simulink model "CSRT_NL"  (R2020b)
settings: Solver=FixedStepAuto  StartTime=0.0  StopTime=15  FixedStep=0.01  RelTol=1e-3
values from neighbouring files (symbols this model uses):
  Cafs = 10    [CSTR_PID.m]
  Cas = 8.564    [CSTR_PID.m]
  dCafs = 0    [CSTR_PID.m]
  dTfs = 0    [CSTR_PID.m]
  dTjs = 0    [CSTR_PID.m]
  Fs = 1    [CSTR_PID.m]
  Ki1 = Kp1/Ti1    (= 18.4487621431)    [CSTR_PID.m]
  Kp1 = (T/(K*L))*(0.9 + L/(12*T))    (= 5.91300687974)    [CSTR_PID.m]    (also in Exp2_guia.m = 0.469047619048)
  RefCa = 9    [CSTR_PID.m]
  Tfs = 298    [CSTR_PID.m]
  Tjs = 298    [CSTR_PID.m]
  Ts = 311.2    [CSTR_PID.m]
libraries: pid_lib x1
settings Model: Creator=franc  LastModifiedBy=Francinildo Barbosa

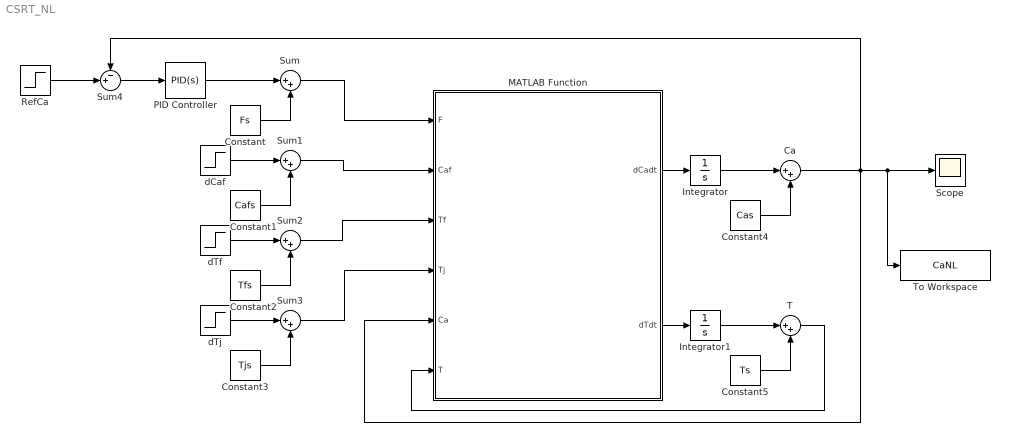
== system CSRT_NL ==
  "              Ca" : Sum  Inputs=|++
  "            T" : Sum  Inputs=|++
  Constant : Constant  Value=Fs
  Constant1 : Constant  Value=Cafs
  Constant2 : Constant  Value=Tfs
  Constant3 : Constant  Value=Tjs
  Constant4 : Constant  Value=Cas
  Constant5 : Constant  Value=Ts
  Integrator : Integrator
  Integrator1 : Integrator
  MATLAB Function : MATLAB Function  TreatAsAtomicUnit=on
  PID Controller : pid_lib/PID Controller  Controller=PID  Form=Parallel  TimeDomain=Continuous-time  UseExternalTs=off  SampleTime=-1  IntegratorMethod=Forward Euler  FilterMethod=Forward Euler  ControllerParametersSource=internal  P=Kp1  I=Ki1  D=0  UseFilter=on  N=100  TunerSelectOption=Transfer Function Based (PID Tuner App)  InitialConditionSource=internal  InitialConditionForIntegrator=0  InitialConditionForFilter=0  DifferentiatorICPrevScaledInput=0  ExternalReset=none  TrackingMode=off  Kt=1  LimitOutput=off  SatLimitsSource=internal  UpperSaturationLimit=inf  LowerSaturationLimit=-inf  LinearizeAsGain=on  AntiWindupMode=none  Kb=1  POutMin=[]  POutMax=[]  IOutMin=[]  IOutMax=[]  DOutMin=[]  DOutMax=[]  NOutMin=[]  NOutMax=[]  SumOutMin=[]  SumOutMax=[]  SaturationOutMin=[]  SaturationOutMax=[]  PParamMin=[]  PParamMax=[]  IParamMin=[]  IParamMax=[]  DParamMin=[]  DParamMax=[]  NParamMin=[]  NParamMax=[]  KbParamMin=[]  KbParamMax=[]  KtParamMin=[]  KtParamMax=[]  KbOutMin=[]  KbOutMax=[]  KtOutMin=[]  KtOutMax=[]  IntegratorOutMin=[]  IntegratorOutMax=[]  FilterOutMin=[]  FilterOutMax=[]  SumI1OutMin=[]  SumI1OutMax=[]  SumI2OutMin=[]  SumI2OutMax=[]  SumI3OutMin=[]  SumI3OutMax=[]  SumI4OutMin=[]  SumI4OutMax=[]  SumDOutMin=[]  SumDOutMax=[]  DifferentiatorOutMin=[]  DifferentiatorOutMax=[]  FilterDiffOutCoefMin=[]  FilterDiffOutCoefMax=[]  ReciprocalOutMin=[]  ReciprocalOutMax=[]  SumDenOutMin=[]  SumDenOutMax=[]  SumNumOutMin=[]  SumNumOutMax=[]  DivideOutMin=[]  DivideOutMax=[]  UdiffTsProdOutMin=[]  UdiffTsProdOutMax=[]  NTsProdOutMin=[]  NTsProdOutMax=[]  UintegralTsProdOutMin=[]  UintegralTsProdOutMax=[]  UngainTsProdOutMin=[]  UngainTsProdOutMax=[]  IntegratorContinuousStateAttributes=''  IntegratorStateMustResolveToSignalObject=off  IntegratorRTWStateStorageClass=Auto  FilterContinuousStateAttributes=''  FilterStateMustResolveToSignalObject=off  FilterRTWStateStorageClass=Auto  ParallelPVariant=InternalParameters  IdealPVariant=Disabled  IVariant=InternalParameters  DVariant=InternalParameters  IntegratorVariant=Continuous  SatVariant=Disabled  AWVariant=Passthrough  PCopyVariant=Disabled  TRVariant=Disabled  FdbkBlocksVariant=Forward  IdealPFdbkVariant=Disabled  SatFdbkVariant=Disabled  DerivativeFilterVariant=ContFilter  NVariant=InternalParameters  NCopyVariant=Disabled  FilterICVariant=InternalICsFilter  IntegratorICVariant=InternalICs  ExternalResetVariant=Disabled  TRSumVariant=Passthrough  SumFdbkVariant=Disabled  SumVariant=Sum_PID  TsampFilterVariant=InternalTs  TsampNgainVariant=Passthrough  TsampIntegralVariant=Passthrough  ExternalSaturationOutDataTypeStr=Inherit: Same as second input
  RefCa : Step  Time=0  After=RefCa  SampleTime=0
  Scope : Scope
  Sum{,1..3} (4 alike) : Sum  Inputs=|++
  Sum4 : Sum  Inputs=-+|
  To Workspace : ToWorkspace  VariableName=CaNL  SaveFormat=Timeseries  SampleTime=-1
  dCaf : Step  Time=0  After=dCafs  SampleTime=0
  dTf : Step  Time=0  After=dTfs  SampleTime=0
  dTj : Step  Time=0  After=dTjs  SampleTime=0
  wires:
  Constant/1 -> Sum/2
  Sum/1 -> MATLAB Function/1(F)
  Constant1/1 -> Sum1/2
  dCaf/1 -> Sum1/1
  Sum1/1 -> MATLAB Function/2(Caf)
  Constant2/1 -> Sum2/2
  dTf/1 -> Sum2/1
  Sum2/1 -> MATLAB Function/3(Tf)
  dTj/1 -> Sum3/1
  Constant3/1 -> Sum3/2
  Sum3/1 -> MATLAB Function/4(Tj)
  Integrator/1 -> "              Ca"/1
  MATLAB Function/1(dCadt) -> Integrator/1
  Constant4/1 -> "              Ca"/2
  "              Ca"/1 -> Sum4/1, MATLAB Function/5(Ca), To Workspace/1, Scope/1
  MATLAB Function/2(dTdt) -> Integrator1/1
  Integrator1/1 -> "            T"/1
  Constant5/1 -> "            T"/2
  "            T"/1 -> MATLAB Function/6(T)
  PID Controller/1 -> Sum/1
  Sum4/1 -> PID Controller/1
  RefCa/1 -> Sum4/2

== matlab function CSRT_NL/MATLAB Function ==
  data: F input; dCadt output; dTdt output; Caf input; Tf input; Tj input; Ca input; T input
function [dCadt, dTdt] = fcn(F, Caf, Tf, Tj, Ca, T)
% Definição dos parâmetros do reator
V     = 1;         % Volume do reator (m^3)
dE    = 11843;     % Energia de ativação (J/mol)
rhocp = 500;       % Densidade*Capacidade térmica (J/(K*m^3))
R     = 1.987;     % Constante de gás ideal (L/(mol*K))
UA    = 150;       % Coef. geral transf. calor*área para troca de calor (J/(Kh))
k0    = 9703*3600; % Fator pré-exponencial (h^-1)
dH    = -5960;     % Calor de reação (J/mol)

r = k0*exp(-dE/(R*T))*Ca;

dCadt = (F/V)*(Caf - Ca) - r;
dTdt  = (F/V)*(Tf - T) + (-dH/rhocp)*r - (UA/(V*rhocp))*(T - Tj);
